simulink model "lic_old"  (R2021b)
settings: Solver=VariableStepAuto  StartTime=0.0  StopTime=10.0  RelTol=1e-3
undefined symbols (not defined in the file): C_TICK_TIME_S, ENUM_LANEQUALITY_HIGH, ENUM_LANEQUALITY_MEDIUM, ENUM_LFCSTATE_DEGRADED, FALSE, KAPP_VehicleWidth_m, KIFO_C1Max4Act_rad, KIFO_C2Max4Act_rat, KIFO_C2Max4Disable_rat, KIFO_C2Max4DisableThr_s, KIFO_Lane4ActThr_s, KIFO_LaneWidthLowThr_m, KIFO_LaneWidthUpThr_m, KIFO_TLCTriggerThrHysis_s, KPER_C0CrossingThr_m, KPER_CalDefaultTLC_s, KPER_CalTLCMax_s, KPER_CalTLCMin_s, KPER_DefaultLaneWidth_m, KPER_LaneWidHoldOnTime_s, KPER_LaneWidRampFinErrThres_m, KPER_LaneWidRampFinTimeThres_s, KPER_LaneWidRampInFalRt_mps, KPER_LaneWidRampInRisRt_mps, KPER_LaneWidRampOutFalRt_mps, KPER_LaneWidRampOutRisRt_mps, KPER_TLCDefaultValue_s, KPER_UseCalTLC_flg, MIFO_TLCThr4LKA_s, TRUE
libraries: hcu_lib x33, simulink x8
(part 2 of 2)

== system lic_old/Lane_Process/LaneCalculation/GenerateLeftLane ==
  VDINR_LaneC0L_m : Inport
  VLIC_EstLaneC0L_m : Inport  Port=2
  VDINR_LaneC1L_rad : Inport  Port=3
  VLIC_EstLaneC1L_rad : Inport  Port=4
  VDINR_LaneC2L_rat : Inport  Port=5
  VLIC_EstLaneC2L_rat : Inport  Port=6
  VDINR_LaneC3L_rat : Inport  Port=7
  VLIC_EstLaneC3L_rat : Inport  Port=8
  VLIC_LeftLaneAvail_flg : Inport  Port=9
  Switch{3,12..14} (4 alike) : Switch  Criteria=u2 ~= 0
  VLIC_LaneC0L_m : Outport
  VLIC_LaneC1L_rad : Outport  Port=2
  VLIC_LaneC2L_rat : Outport  Port=3
  VLIC_LaneC3L_rat : Outport  Port=4
  wires:
  Switch14/1 -> VLIC_LaneC3L_rat/1  "VLIC_LaneC3L_rat"
  VDINR_LaneC0L_m/1 -> Switch3/1
  VDINR_LaneC3L_rat/1 -> Switch14/1
  VLIC_EstLaneC3L_rat/1 -> Switch14/3
  VLIC_LeftLaneAvail_flg/1 -> Switch3/2, Switch12/2, Switch13/2, Switch14/2
  VDINR_LaneC2L_rat/1 -> Switch13/1
  VLIC_EstLaneC2L_rat/1 -> Switch13/3
  Switch13/1 -> VLIC_LaneC2L_rat/1  "VLIC_LaneC2L_rat"
  Switch3/1 -> VLIC_LaneC0L_m/1  "VLIC_LaneC0L_m"
  VDINR_LaneC1L_rad/1 -> Switch12/1
  VLIC_EstLaneC1L_rad/1 -> Switch12/3
  Switch12/1 -> VLIC_LaneC1L_rad/1  "VLIC_LaneC1L_rad"
  VLIC_EstLaneC0L_m/1 -> Switch3/3

== system lic_old/Lane_Process/LaneCalculation/GenerateRightLane ==
  VDINR_LaneC0R_m : Inport
  VLIC_EstLaneC0R_m : Inport  Port=2
  VDINR_LaneC1R_rad : Inport  Port=3
  VLIC_EstLaneC1R_rad : Inport  Port=4
  VDINR_LaneC2R_rat : Inport  Port=5
  VLIC_EstLaneC2R_rat : Inport  Port=6
  VDINR_LaneC3R_rat : Inport  Port=7
  VLIC_EstLaneC3R_rat : Inport  Port=8
  VLIC_RightLaneAvail_flg : Inport  Port=9
  Switch{3,12..14} (4 alike) : Switch  Criteria=u2 ~= 0
  VLIC_LaneC0R_m : Outport
  VLIC_LaneC1R_rad : Outport  Port=2
  VLIC_LaneC2R_rat : Outport  Port=3
  VLIC_LaneC3R_rat : Outport  Port=4
  wires:
  VLIC_EstLaneC0R_m/1 -> Switch3/3
  Switch12/1 -> VLIC_LaneC1R_rad/1  "VLIC_LaneC1R_rad"
  VLIC_EstLaneC1R_rad/1 -> Switch12/3
  VDINR_LaneC1R_rad/1 -> Switch12/1
  Switch3/1 -> VLIC_LaneC0R_m/1  "VLIC_LaneC0R_m"
  Switch13/1 -> VLIC_LaneC2R_rat/1  "VLIC_LaneC2R_rat"
  VLIC_EstLaneC2R_rat/1 -> Switch13/3
  VDINR_LaneC2R_rat/1 -> Switch13/1
  VLIC_RightLaneAvail_flg/1 -> Switch14/2, Switch13/2, Switch12/2, Switch3/2
  Switch14/1 -> VLIC_LaneC3R_rat/1  "VLIC_LaneC3R_rat"
  VLIC_EstLaneC3R_rat/1 -> Switch14/3
  VDINR_LaneC3R_rat/1 -> Switch14/1
  VDINR_LaneC0R_m/1 -> Switch3/1

== system lic_old/Lane_Process/LaneCalculation/LR_Available ==
  VDINR_LaneC0L_m : Inport
  VDINR_LaneC0R_m : Inport  Port=2
  VDINR_LaneC1L_rad : Inport  Port=3
  VDINR_LaneC1R_rad : Inport  Port=4
  VDINR_LaneC2L_rat : Inport  Port=5
  VDINR_LaneC2R_rat : Inport  Port=6
  VDINR_LaneC3L_rat : Inport  Port=7
  VDINR_LaneC3R_rat : Inport  Port=8
  Enable : EnablePort  StatesWhenEnabling=reset
  Add{,1..3} (4 alike) : Sum
  Gain{,1..3} (4 alike) : Gain  Gain=0.5
  VLIC_RLCenterLineC0_m : Outport
  VLIC_RLCenterLineC1_rad : Outport  Port=2
  VLIC_RLCenterLineC2_rat : Outport  Port=3
  VLIC_RLCenterLineC3_rat : Outport  Port=4
  wires:
  Gain3/1 -> VLIC_RLCenterLineC3_rat/1  "VLIC_RLCenterLineC3_rat"
  VDINR_LaneC3R_rat/1 -> Add3/2
  VDINR_LaneC3L_rat/1 -> Add3/1
  Add3/1 -> Gain3/1
  Gain2/1 -> VLIC_RLCenterLineC2_rat/1  "VLIC_RLCenterLineC2_rat"
  VDINR_LaneC2R_rat/1 -> Add2/2
  VDINR_LaneC2L_rat/1 -> Add2/1
  Gain1/1 -> VLIC_RLCenterLineC1_rad/1  "VLIC_RLCenterLineC1_rad"
  Add2/1 -> Gain2/1
  Add1/1 -> Gain1/1
  VDINR_LaneC1R_rad/1 -> Add1/2
  VDINR_LaneC1L_rad/1 -> Add1/1
  Gain/1 -> VLIC_RLCenterLineC0_m/1  "VLIC_RLCenterLineC0_m"
  Add/1 -> Gain/1
  VDINR_LaneC0R_m/1 -> Add/2
  VDINR_LaneC0L_m/1 -> Add/1

== system lic_old/Lane_Process/LaneCalculation/LR_NotAvailable ==
  VLIC_EstLaneC0L_m : Inport
  VLIC_EstLaneC0R_m : Inport  Port=2
  VLIC_EstLaneC1L_rad : Inport  Port=3
  VLIC_EstLaneC1R_rad : Inport  Port=4
  VLIC_EstLaneC2L_rat : Inport  Port=5
  VLIC_EstLaneC2R_rat : Inport  Port=6
  VLIC_EstLaneC3L_rat : Inport  Port=7
  VLIC_EstLaneC3R_rat : Inport  Port=8
  Enable : EnablePort  StatesWhenEnabling=reset
  Add{,1..3} (4 alike) : Sum
  Gain{,1..3} (4 alike) : Gain  Gain=0.5
  VLIC_EstCenterLineC0_m : Outport
  VLIC_EstCenterLineC1_rad : Outport  Port=2
  VLIC_EstCenterLineC2_rat : Outport  Port=3
  VLIC_EstCenterLineC3_rat : Outport  Port=4
  wires:
  Gain3/1 -> VLIC_EstCenterLineC3_rat/1  "VLIC_EstCenterLineC3_rat"
  VLIC_EstLaneC3R_rat/1 -> Add3/2
  VLIC_EstLaneC3L_rat/1 -> Add3/1
  Add3/1 -> Gain3/1
  Gain2/1 -> VLIC_EstCenterLineC2_rat/1  "VLIC_EstCenterLineC2_rat"
  VLIC_EstLaneC2R_rat/1 -> Add2/2
  VLIC_EstLaneC2L_rat/1 -> Add2/1
  Gain1/1 -> VLIC_EstCenterLineC1_rad/1  "VLIC_EstCenterLineC1_rad"
  Add2/1 -> Gain2/1
  Add1/1 -> Gain1/1
  VLIC_EstLaneC1R_rad/1 -> Add1/2
  VLIC_EstLaneC1L_rad/1 -> Add1/1
  Gain/1 -> VLIC_EstCenterLineC0_m/1  "VLIC_EstCenterLineC0_m"
  Add/1 -> Gain/1
  VLIC_EstLaneC0R_m/1 -> Add/2
  VLIC_EstLaneC0L_m/1 -> Add/1

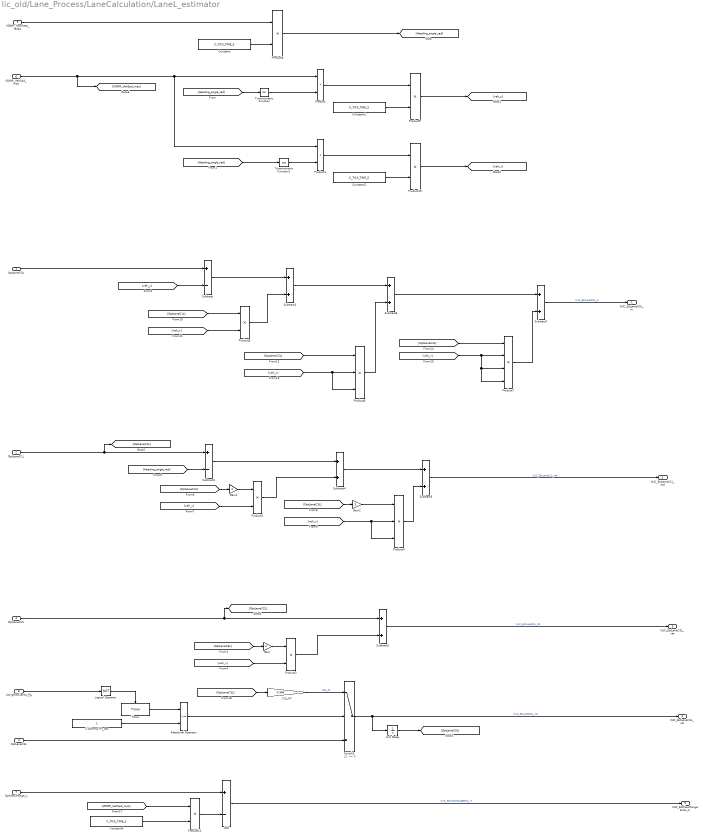
== system lic_old/Lane_Process/LaneCalculation/LaneL_estimator ==
  OptLaneC0L : Inport
  OptLaneC1L : Inport  Port=2
  OptLaneC2L : Inport  Port=3
  OptLaneC3L : Inport  Port=4
  VDINR_YawRate_radps : Inport  Port=5
  VDINR_VehSpd_mps : Inport  Port=6
  OptViewRange_L : Inport  Port=7
  UsingRawLaneL_flg : Inport  Port=8
  Add : Sum  Inputs=+-
  C3LRampThr_sec : Constant  OutDataTypeStr=single
  C3L_FF : Gain  Gain=0.994
  Constant{,1..2,4} (4 alike) : Constant  Value=C_TICK_TIME_S
  Gain : Gain  Gain=3
  Gain1 : Gain  Gain=2
  Gain2 : Gain  Gain=3
  Logical Operator : Logic  Operator=NOT  AllPortsSameDT=off  OutDataTypeStr=boolean
  Product{,1..3,5,8..10,12} (9 alike) : Product
  Product4 : Product  Inputs=3
  Product6 : Product  Inputs=3
  Product7 : Product  Inputs=4
  Relational Operator : RelationalOperator  OutDataTypeStr=boolean  RndMeth=Nearest
  Subtract : Sum  Inputs=+-
  Subtract{1..2,4..7} (6 alike) : Sum
  Subtract3 : Sum  Inputs=+-
  Switch2 : Switch  Criteria=u2 ~= 0
  Timer : hcu_lib/Timer  SystemSampleTime=-1  VariantActivationTime=update diagram  Latency=0  AutoFrameSizeCalculation=off
  Trigonometric Function : Trigonometry
  Trigonometric Function1 : Trigonometry  Operator=cos
  Unit Delay : UnitDelay  SampleTime=-1  HasFrameUpgradeWarning=on
  VLIC_EstLaneC0L_m : Outport
  VLIC_EstLaneC1L_rad : Outport  Port=2
  VLIC_EstLaneC2L_rat : Outport  Port=3
  VLIC_EstLaneC3L_rat : Outport  Port=4
  VLIC_EstViewRangeEndL_m : Outport  Port=5
  wires:
  Product8/1 -> [Heading_angle_rad]
  Unit Delay/1 -> [OptLaneC3L]
  Logical Operator/1 -> Timer/Enable
  C3L_FF/1 -> Switch2/1  "C3L_FF"
  [OptLaneC3L] -> C3L_FF/1
  Switch2/1 -> VLIC_EstLaneC3L_rat/1, Unit Delay/1  "VLIC_EstLaneC3L_rat"
  OptLaneC3L/1 -> Switch2/3
  Relational Operator/1 -> Switch2/2
  C3LRampThr_sec/1 -> Relational Operator/2
  Timer/1 -> Relational Operator/1
  UsingRawLaneL_flg/1 -> Logical Operator/1
  Constant4/1 -> Product12/2
  Add/1 -> VLIC_EstViewRangeEndL_m/1  "VLIC_EstViewRangeEndL_m"
  Product12/1 -> Add/2
  [VDINR_VehSpd_mps] -> Product12/1
  OptViewRange_L/1 -> Add/1
  VDINR_YawRate_radps/1 -> Product8/1
  Product1/1 -> Product10/1
  Constant2/1 -> Product10/2
  Product/1 -> Product9/1
  Constant1/1 -> Product9/2
  Constant/1 -> Product8/2
  Subtract7/1 -> VLIC_EstLaneC0L_m/1  "VLIC_EstLaneC0L_m"
  Product7/1 -> Subtract7/2
  [veh_x] -> Product7/3, Product7/4, Product7/2
  [OptLaneC3L] -> Product7/1
  Subtract6/1 -> Subtract7/1
  Product6/1 -> Subtract6/2
  [veh_x] -> Product6/3, Product6/2
  [OptLaneC2L] -> Product6/1
  Subtract1/1 -> Subtract6/1
  Product5/1 -> Subtract1/2
  [veh_x] -> Product5/2
  [OptLaneC1L] -> Product5/1
  Subtract5/1 -> VLIC_EstLaneC1L_rad/1  "VLIC_EstLaneC1L_rad"
  Product4/1 -> Subtract5/2
  [veh_x] -> Product4/2, Product4/3
  Gain2/1 -> Product4/1
  [OptLaneC3L] -> Gain2/1
  Subtract4/1 -> Subtract5/1
  Product3/1 -> Subtract4/2
  [veh_x] -> Product3/2
  Gain1/1 -> Product3/1
  [OptLaneC2L] -> Gain1/1
  Subtract3/1 -> Subtract4/1
  [Heading_angle_rad] -> Subtract3/2
  OptLaneC1L/1 -> Subtract3/1, [OptLaneC1L]
  Subtract2/1 -> VLIC_EstLaneC2L_rat/1  "VLIC_EstLaneC2L_rat"
  [veh_x] -> Product2/2
  Gain/1 -> Product2/1
  [OptLaneC3L] -> Gain/1
  Product2/1 -> Subtract2/2
  OptLaneC2L/1 -> Subtract2/1, [OptLaneC2L]
  Subtract/1 -> Subtract1/1
  [veh_y] -> Subtract/2
  OptLaneC0L/1 -> Subtract/1
  Product10/1 -> [veh_x]
  Trigonometric Function1/1 -> Product1/2
  [Heading_angle_rad] -> Trigonometric Function1/1
  Product9/1 -> [veh_y]
  Trigonometric Function/1 -> Product/2
  [Heading_angle_rad] -> Trigonometric Function/1
  VDINR_VehSpd_mps/1 -> Product/1, Product1/1, [VDINR_VehSpd_mps]

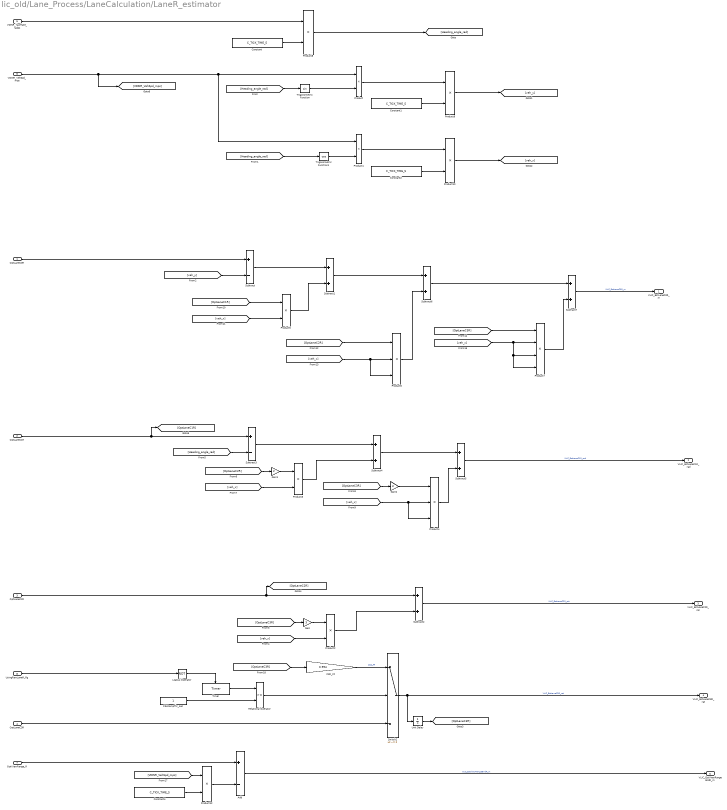
== system lic_old/Lane_Process/LaneCalculation/LaneR_estimator ==
  OptLaneC0R : Inport
  OptLaneC1R : Inport  Port=2
  OptLaneC2R : Inport  Port=3
  OptLaneC3R : Inport  Port=4
  VDINR_YawRate_radps : Inport  Port=5
  VDINR_VehSpd_mps : Inport  Port=6
  OptViewRange_R : Inport  Port=7
  UsingRawLaneR_flg : Inport  Port=8
  Add : Sum  Inputs=+-
  C3LRampThr_sec : Constant  OutDataTypeStr=single
  C3R_FF : Gain  Gain=0.994
  Constant{,1..2,4} (4 alike) : Constant  Value=C_TICK_TIME_S
  Gain : Gain  Gain=3
  Gain1 : Gain  Gain=2
  Gain2 : Gain  Gain=3
  Logical Operator : Logic  Operator=NOT  AllPortsSameDT=off  OutDataTypeStr=boolean
  Product{,1..3,5,8..10,12} (9 alike) : Product
  Product4 : Product  Inputs=3
  Product6 : Product  Inputs=3
  Product7 : Product  Inputs=4
  Relational Operator : RelationalOperator  OutDataTypeStr=boolean  RndMeth=Nearest
  Subtract : Sum  Inputs=+-
  Subtract{1..2,4..7} (6 alike) : Sum
  Subtract3 : Sum  Inputs=+-
  Switch2 : Switch  Criteria=u2 ~= 0
  Timer : hcu_lib/Timer  SystemSampleTime=-1  VariantActivationTime=update diagram  Latency=0  AutoFrameSizeCalculation=off
  Trigonometric Function : Trigonometry
  Trigonometric Function1 : Trigonometry  Operator=cos
  Unit Delay : UnitDelay  SampleTime=-1  HasFrameUpgradeWarning=on
  VLIC_EstLaneC0R_m : Outport
  VLIC_EstLaneC1R_rad : Outport  Port=2
  VLIC_EstLaneC2R_rat : Outport  Port=3
  VLIC_EstLaneC3R_rat : Outport  Port=4
  VLIC_EstViewRangeEndR_m : Outport  Port=5
  wires:
  Unit Delay/1 -> [OptLaneC3R]
  Logical Operator/1 -> Timer/Enable
  OptLaneC3R/1 -> Switch2/3
  C3R_FF/1 -> Switch2/1  "C3R_FF"
  [OptLaneC3R] -> C3R_FF/1
  Switch2/1 -> VLIC_EstLaneC3R_rat/1, Unit Delay/1  "VLIC_EstLaneC3R_rat"
  Relational Operator/1 -> Switch2/2
  C3LRampThr_sec/1 -> Relational Operator/2
  Timer/1 -> Relational Operator/1
  UsingRawLaneR_flg/1 -> Logical Operator/1
  VDINR_VehSpd_mps/1 -> [VDINR_VehSpd_mps], Product1/1, Product/1
  [Heading_angle_rad] -> Trigonometric Function/1
  Trigonometric Function/1 -> Product/2
  Product9/1 -> [veh_y]
  [Heading_angle_rad] -> Trigonometric Function1/1
  Trigonometric Function1/1 -> Product1/2
  Product10/1 -> [veh_x]
  OptLaneC0R/1 -> Subtract/1
  [veh_y] -> Subtract/2
  Subtract/1 -> Subtract1/1
  OptLaneC2R/1 -> [OptLaneC2R], Subtract2/1
  Product2/1 -> Subtract2/2
  [OptLaneC3R] -> Gain/1
  Gain/1 -> Product2/1
  [veh_x] -> Product2/2
  Subtract2/1 -> VLIC_EstLaneC2R_rat/1  "VLIC_EstLaneC2R_rat"
  OptLaneC1R/1 -> [OptLaneC1R], Subtract3/1
  [Heading_angle_rad] -> Subtract3/2
  Subtract3/1 -> Subtract4/1
  [OptLaneC2R] -> Gain1/1
  Gain1/1 -> Product3/1
  [veh_x] -> Product3/2
  Product3/1 -> Subtract4/2
  Subtract4/1 -> Subtract5/1
  [OptLaneC3R] -> Gain2/1
  Gain2/1 -> Product4/1
  [veh_x] -> Product4/3, Product4/2
  Product4/1 -> Subtract5/2
  Subtract5/1 -> VLIC_EstLaneC1R_rad/1  "VLIC_EstLaneC1R_rad"
  [OptLaneC1R] -> Product5/1
  [veh_x] -> Product5/2
  Product5/1 -> Subtract1/2
  Subtract1/1 -> Subtract6/1
  [OptLaneC2R] -> Product6/1
  [veh_x] -> Product6/2, Product6/3
  Product6/1 -> Subtract6/2
  Subtract6/1 -> Subtract7/1
  [OptLaneC3R] -> Product7/1
  [veh_x] -> Product7/2, Product7/4, Product7/3
  Product7/1 -> Subtract7/2
  Subtract7/1 -> VLIC_EstLaneC0R_m/1  "VLIC_EstLaneC0R_m"
  Constant/1 -> Product8/2
  Constant1/1 -> Product9/2
  Product/1 -> Product9/1
  Constant2/1 -> Product10/2
  Product1/1 -> Product10/1
  VDINR_YawRate_radps/1 -> Product8/1
  Product8/1 -> [Heading_angle_rad]
  OptViewRange_R/1 -> Add/1
  [VDINR_VehSpd_mps] -> Product12/1
  Constant4/1 -> Product12/2
  Product12/1 -> Add/2
  Add/1 -> VLIC_EstViewRangeEndR_m/1  "VLIC_EstViewRangeEndR_m"

== system lic_old/Lane_Process/LaneCalculation/LaneResidual_Calculation ==
  VLIC_EstViewRangeEndL_m : Inport
  VDINR_VehSpd_mps : Inport  Port=2
  VLIC_EstViewRangeEndR_m : Inport  Port=3
  Constant6 : Constant  Value=3  OutDataTypeStr=single
  Constant7 : Constant  Value=3  OutDataTypeStr=single
  Saturation1 : Saturate  UpperLimit=3  LowerLimit=0
      settings: AttributesFormatString=upper = %<UpperLimit>\nlower = %<LowerLimit>
  Saturation2 : Saturate  UpperLimit=3  LowerLimit=0
      settings: AttributesFormatString=upper = %<UpperLimit>\nlower = %<LowerLimit>
  divide : hcu_lib/divide
  divide1 : hcu_lib/divide
  VLIC_ResidualLaneL_s : Outport
  VLIC_ResidualLaneR_s : Outport  Port=2
  wires:
  Saturation2/1 -> VLIC_ResidualLaneR_s/1  "VLIC_ResidualLaneR_s"
  Saturation1/1 -> VLIC_ResidualLaneL_s/1  "VLIC_ResidualLaneL_s"
  divide1/1 -> Saturation2/1
  Constant7/1 -> divide1/3
  VDINR_VehSpd_mps/1 -> divide/2, divide1/2
  VLIC_EstViewRangeEndR_m/1 -> divide1/1
  Constant6/1 -> divide/3
  VLIC_EstViewRangeEndL_m/1 -> divide/1
  divide/1 -> Saturation1/1

== system lic_old/Lane_Process/LaneCalculation/LaneWidth ==
  VLIC_LeftLaneAvail_flg : Inport
  VLIC_RightLaneAvail_flg : Inport  Port=2
  VLIC_LaneC0L_m : Inport  Port=3
  VLIC_LaneC0R_m : Inport  Port=4
  Add : Sum  Inputs=+-
  Delay : Delay  DelayLength=1  InitialCondition=KPER_DefaultLaneWidth_m
  KPER_DefaultLaneWidth_m : Constant  Value=KPER_DefaultLaneWidth_m
  KPER_LaneWidHoldOnTime_s : Constant  Value=KPER_LaneWidHoldOnTime_s
  KPER_LaneWidRampFinErrThres_m : Constant  Value=KPER_LaneWidRampFinErrThres_m
  KPER_LaneWidRampFinTimeThres_s : Constant  Value=KPER_LaneWidRampFinTimeThres_s
  KPER_LaneWidRampInFalRt_mps : Constant  Value=KPER_LaneWidRampInFalRt_mps
  KPER_LaneWidRampInRisRt_mps : Constant  Value=KPER_LaneWidRampInRisRt_mps
  KPER_LaneWidRampOutFalRt_mps : Constant  Value=KPER_LaneWidRampOutFalRt_mps
  KPER_LaneWidRampOutRisRt_mps : Constant  Value=KPER_LaneWidRampOutRisRt_mps
  Logical Operator : Logic  Operator=OR  AllPortsSameDT=off  OutDataTypeStr=boolean
  Logical Operator1 : Logic  Operator=NOT  AllPortsSameDT=off  OutDataTypeStr=boolean
  Logical Operator2 : Logic  Operator=NOT  AllPortsSameDT=off  OutDataTypeStr=boolean
  RampInRampOut : hcu_lib/RampInRampOut  SystemSampleTime=-1  VariantActivationTime=update diagram  Latency=0  AutoFrameSizeCalculation=off
  Relational Operator2 : RelationalOperator  OutDataTypeStr=boolean  RndMeth=Nearest
  Switch2 : Switch  Criteria=u2 ~= 0
  Timer : hcu_lib/Timer  SystemSampleTime=-1  VariantActivationTime=update diagram  Latency=0  AutoFrameSizeCalculation=off
  VLIC_LaneWidth_m : Outport
  wires:
  VLIC_RightLaneAvail_flg/1 -> Logical Operator2/1
  VLIC_LeftLaneAvail_flg/1 -> Logical Operator1/1
  KPER_LaneWidHoldOnTime_s/1 -> Relational Operator2/2
  Timer/1 -> Relational Operator2/1
  Relational Operator2/1 -> RampInRampOut/3
  RampInRampOut/1 -> VLIC_LaneWidth_m/1, Delay/1  "VLIC_LaneWidth_m"
  KPER_LaneWidRampFinTimeThres_s/1 -> RampInRampOut/9
  KPER_LaneWidRampFinErrThres_m/1 -> RampInRampOut/8
  KPER_LaneWidRampOutRisRt_mps/1 -> RampInRampOut/6
  KPER_LaneWidRampOutFalRt_mps/1 -> RampInRampOut/7
  KPER_LaneWidRampInFalRt_mps/1 -> RampInRampOut/5
  KPER_LaneWidRampInRisRt_mps/1 -> RampInRampOut/4
  Logical Operator/1 -> Timer/Enable, Switch2/2
  KPER_DefaultLaneWidth_m/1 -> RampInRampOut/2
  Delay/1 -> Switch2/1
  Switch2/1 -> RampInRampOut/1
  Logical Operator1/1 -> Logical Operator/1
  Logical Operator2/1 -> Logical Operator/2
  VLIC_LaneC0L_m/1 -> Add/1
  Add/1 -> Switch2/3
  VLIC_LaneC0R_m/1 -> Add/2

== system lic_old/Lane_Process/LaneCalculation/OnlyL_Available ==
  VLIC_LaneWidth_m : Inport
  VDINR_LaneC0L_m : Inport  Port=2
  VDINR_LaneC1L_rad : Inport  Port=3
  VDINR_LaneC2L_rat : Inport  Port=4
  VDINR_LaneC3L_rat : Inport  Port=5
  Enable : EnablePort  StatesWhenEnabling=reset
  Add : Sum  Inputs=-+
  Add1 : Sum
  Data Type Conversion : DataTypeConversion  OutDataTypeStr=single
  Data Type Conversion1 : DataTypeConversion  OutDataTypeStr=single
  Data Type Conversion2 : DataTypeConversion  OutDataTypeStr=single
  Gain : Gain  Gain=0.5
  VLIC_LCenterLineC0_m : Outport
  VLIC_LCenterLineC1_rad : Outport  Port=2
  VLIC_LCenterLineC2_rat : Outport  Port=3
  VLIC_LCenterLineC3_rat : Outport  Port=4
  wires:
  Data Type Conversion/1 -> VLIC_LCenterLineC1_rad/1  "VLIC_LCenterLineC1_rad"
  Data Type Conversion2/1 -> VLIC_LCenterLineC3_rat/1  "VLIC_LCenterLineC3_rat"
  Data Type Conversion1/1 -> VLIC_LCenterLineC2_rat/1  "VLIC_LCenterLineC2_rat"
  Gain/1 -> VLIC_LCenterLineC0_m/1  "VLIC_LCenterLineC0_m"
  Add1/1 -> Gain/1
  Add/1 -> Add1/1
  VDINR_LaneC3L_rat/1 -> Data Type Conversion2/1
  VDINR_LaneC2L_rat/1 -> Data Type Conversion1/1
  VDINR_LaneC0L_m/1 -> Add/2, Add1/2
  VLIC_LaneWidth_m/1 -> Add/1
  VDINR_LaneC1L_rad/1 -> Data Type Conversion/1

== system lic_old/Lane_Process/LaneCalculation/OnlyR_Available ==
  VLIC_LaneWidth_m : Inport
  VDINR_LaneC0R_m : Inport  Port=2
  VDINR_LaneC1R_rad : Inport  Port=3
  VDINR_LaneC2R_rat : Inport  Port=4
  VDINR_LaneC3R_rat : Inport  Port=5
  Enable : EnablePort  StatesWhenEnabling=reset
  Add : Sum
  Add1 : Sum
  Data Type Conversion : DataTypeConversion  OutDataTypeStr=single
  Data Type Conversion1 : DataTypeConversion  OutDataTypeStr=single
  Data Type Conversion2 : DataTypeConversion  OutDataTypeStr=single
  Gain : Gain  Gain=0.5
  VLIC_RCenterLineC0_m : Outport
  VLIC_RCenterLineC1_rad : Outport  Port=2
  VLIC_RCenterLineC2_rat : Outport  Port=3
  VLIC_RCenterLineC3_rat : Outport  Port=4
  wires:
  Data Type Conversion2/1 -> VLIC_RCenterLineC3_rat/1  "VLIC_RCenterLineC3_rat"
  Data Type Conversion1/1 -> VLIC_RCenterLineC2_rat/1  "VLIC_RCenterLineC2_rat"
  Data Type Conversion/1 -> VLIC_RCenterLineC1_rad/1  "VLIC_RCenterLineC1_rad"
  Gain/1 -> VLIC_RCenterLineC0_m/1  "VLIC_RCenterLineC0_m"
  Add1/1 -> Gain/1
  Add/1 -> Add1/1
  VDINR_LaneC1R_rad/1 -> Data Type Conversion/1
  VLIC_LaneWidth_m/1 -> Add/1
  VDINR_LaneC0R_m/1 -> Add/2, Add1/2
  VDINR_LaneC2R_rat/1 -> Data Type Conversion1/1
  VDINR_LaneC3R_rat/1 -> Data Type Conversion2/1

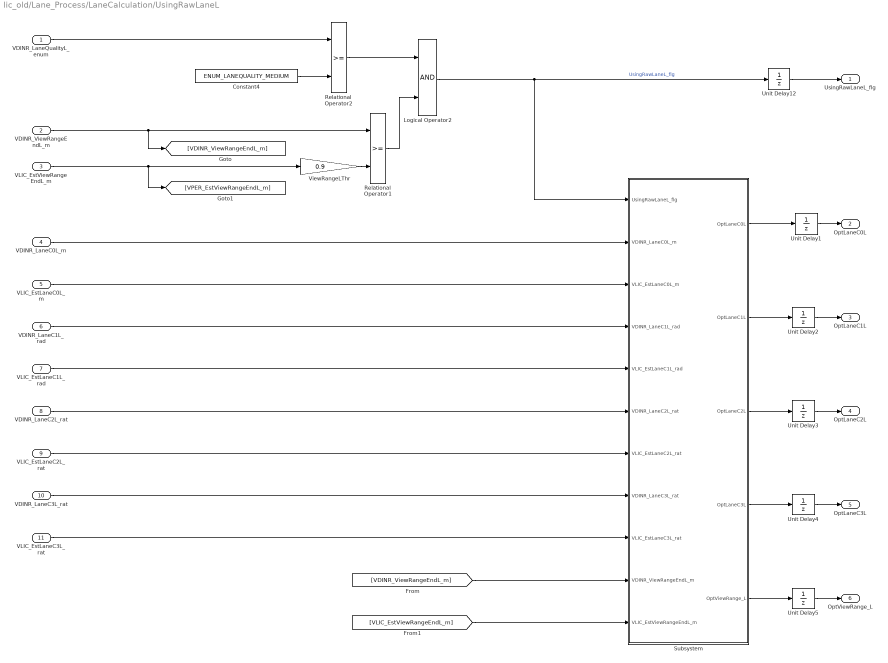
== system lic_old/Lane_Process/LaneCalculation/UsingRawLaneL ==
  VDINR_LaneQualityL_enum : Inport
  VDINR_ViewRangeEndL_m : Inport  Port=2
  VLIC_EstViewRangeEndL_m : Inport  Port=3
  VDINR_LaneC0L_m : Inport  Port=4
  VLIC_EstLaneC0L_m : Inport  Port=5
  VDINR_LaneC1L_rad : Inport  Port=6
  VLIC_EstLaneC1L_rad : Inport  Port=7
  VDINR_LaneC2L_rat : Inport  Port=8
  VLIC_EstLaneC2L_rat : Inport  Port=9
  VDINR_LaneC3L_rat : Inport  Port=10
  VLIC_EstLaneC3L_rat : Inport  Port=11
  Constant4 : Constant  Value=ENUM_LANEQUALITY_MEDIUM
  Logical Operator2 : Logic  AllPortsSameDT=off  OutDataTypeStr=boolean
  Relational Operator1 : RelationalOperator  OutDataTypeStr=boolean  RndMeth=Nearest
  Relational Operator2 : RelationalOperator  OutDataTypeStr=boolean  RndMeth=Nearest
  Subsystem : Subsystem
  Unit Delay{1..5,12} (6 alike) : UnitDelay  SampleTime=-1  HasFrameUpgradeWarning=on
  ViewRangeLThr : Gain  Gain=0.9
  UsingRawLaneL_flg : Outport
  OptLaneC0L : Outport  Port=2
  OptLaneC1L : Outport  Port=3
  OptLaneC2L : Outport  Port=4
  OptLaneC3L : Outport  Port=5
  OptViewRange_L : Outport  Port=6
  wires:
  Subsystem/5(OptViewRange_L) -> Unit Delay5/1
  Subsystem/4(OptLaneC3L) -> Unit Delay4/1
  Subsystem/3(OptLaneC2L) -> Unit Delay3/1
  Subsystem/2(OptLaneC1L) -> Unit Delay2/1
  Subsystem/1(OptLaneC0L) -> Unit Delay1/1
  [VDINR_ViewRangeEndL_m] -> Subsystem/10(VDINR_ViewRangeEndL_m)
  [VLIC_EstViewRangeEndL_m] -> Subsystem/11(VLIC_EstViewRangeEndL_m)
  VLIC_EstLaneC3L_rat/1 -> Subsystem/9(VLIC_EstLaneC3L_rat)
  VDINR_LaneC3L_rat/1 -> Subsystem/8(VDINR_LaneC3L_rat)
  VLIC_EstLaneC2L_rat/1 -> Subsystem/7(VLIC_EstLaneC2L_rat)
  VDINR_LaneC2L_rat/1 -> Subsystem/6(VDINR_LaneC2L_rat)
  VLIC_EstLaneC1L_rad/1 -> Subsystem/5(VLIC_EstLaneC1L_rad)
  VDINR_LaneC1L_rad/1 -> Subsystem/4(VDINR_LaneC1L_rad)
  VLIC_EstLaneC0L_m/1 -> Subsystem/3(VLIC_EstLaneC0L_m)
  VDINR_LaneC0L_m/1 -> Subsystem/2(VDINR_LaneC0L_m)
  Logical Operator2/1 -> Unit Delay12/1, Subsystem/1(UsingRawLaneL_flg)  "UsingRawLaneL_flg"
  VDINR_LaneQualityL_enum/1 -> Relational Operator2/1
  Constant4/1 -> Relational Operator2/2
  Relational Operator2/1 -> Logical Operator2/1
  VDINR_ViewRangeEndL_m/1 -> Relational Operator1/1, [VDINR_ViewRangeEndL_m]
  VLIC_EstViewRangeEndL_m/1 -> ViewRangeLThr/1, [VPER_EstViewRangeEndL_m]
  ViewRangeLThr/1 -> Relational Operator1/2
  Relational Operator1/1 -> Logical Operator2/2
  Unit Delay12/1 -> UsingRawLaneL_flg/1
  Unit Delay1/1 -> OptLaneC0L/1
  Unit Delay2/1 -> OptLaneC1L/1
  Unit Delay3/1 -> OptLaneC2L/1
  Unit Delay4/1 -> OptLaneC3L/1
  Unit Delay5/1 -> OptViewRange_L/1

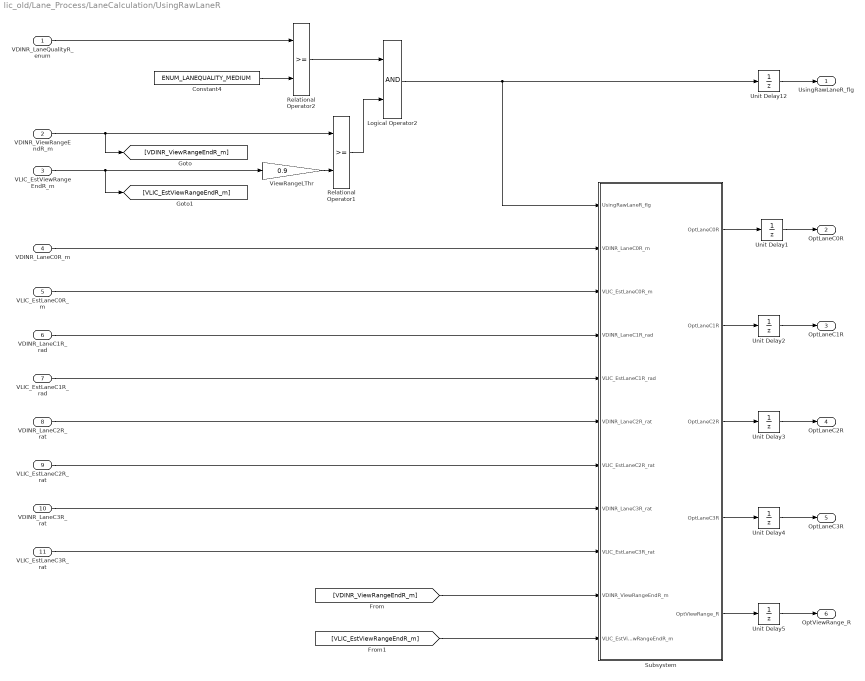
== system lic_old/Lane_Process/LaneCalculation/UsingRawLaneR ==
  VDINR_LaneQualityR_enum : Inport
  VDINR_ViewRangeEndR_m : Inport  Port=2
  VLIC_EstViewRangeEndR_m : Inport  Port=3
  VDINR_LaneC0R_m : Inport  Port=4
  VLIC_EstLaneC0R_m : Inport  Port=5
  VDINR_LaneC1R_rad : Inport  Port=6
  VLIC_EstLaneC1R_rad : Inport  Port=7
  VDINR_LaneC2R_rat : Inport  Port=8
  VLIC_EstLaneC2R_rat : Inport  Port=9
  VDINR_LaneC3R_rat : Inport  Port=10
  VLIC_EstLaneC3R_rat : Inport  Port=11
  Constant4 : Constant  Value=ENUM_LANEQUALITY_MEDIUM
  Logical Operator2 : Logic  AllPortsSameDT=off  OutDataTypeStr=boolean
  Relational Operator1 : RelationalOperator  OutDataTypeStr=boolean  RndMeth=Nearest
  Relational Operator2 : RelationalOperator  OutDataTypeStr=boolean  RndMeth=Nearest
  Subsystem : Subsystem
  Unit Delay{1..5,12} (6 alike) : UnitDelay  SampleTime=-1  HasFrameUpgradeWarning=on
  ViewRangeLThr : Gain  Gain=0.9
  UsingRawLaneR_flg : Outport
  OptLaneC0R : Outport  Port=2
  OptLaneC1R : Outport  Port=3
  OptLaneC2R : Outport  Port=4
  OptLaneC3R : Outport  Port=5
  OptViewRange_R : Outport  Port=6
  wires:
  Subsystem/5(OptViewRange_R) -> Unit Delay5/1
  Subsystem/4(OptLaneC3R) -> Unit Delay4/1
  Subsystem/3(OptLaneC2R) -> Unit Delay3/1
  Subsystem/2(OptLaneC1R) -> Unit Delay2/1
  Subsystem/1(OptLaneC0R) -> Unit Delay1/1
  [VDINR_ViewRangeEndR_m] -> Subsystem/10(VDINR_ViewRangeEndR_m)
  [VLIC_EstViewRangeEndR_m] -> Subsystem/11(VLIC_EstViewRangeEndR_m)
  VLIC_EstLaneC3R_rat/1 -> Subsystem/9(VLIC_EstLaneC3R_rat)
  VDINR_LaneC3R_rat/1 -> Subsystem/8(VDINR_LaneC3R_rat)
  VLIC_EstLaneC2R_rat/1 -> Subsystem/7(VLIC_EstLaneC2R_rat)
  VDINR_LaneC2R_rat/1 -> Subsystem/6(VDINR_LaneC2R_rat)
  VLIC_EstLaneC1R_rad/1 -> Subsystem/5(VLIC_EstLaneC1R_rad)
  VDINR_LaneC1R_rad/1 -> Subsystem/4(VDINR_LaneC1R_rad)
  VLIC_EstLaneC0R_m/1 -> Subsystem/3(VLIC_EstLaneC0R_m)
  VDINR_LaneC0R_m/1 -> Subsystem/2(VDINR_LaneC0R_m)
  Logical Operator2/1 -> Unit Delay12/1, Subsystem/1(UsingRawLaneR_flg)
  VDINR_LaneQualityR_enum/1 -> Relational Operator2/1
  Constant4/1 -> Relational Operator2/2
  Relational Operator2/1 -> Logical Operator2/1
  VDINR_ViewRangeEndR_m/1 -> Relational Operator1/1, [VDINR_ViewRangeEndR_m]
  VLIC_EstViewRangeEndR_m/1 -> ViewRangeLThr/1, [VLIC_EstViewRangeEndR_m]
  ViewRangeLThr/1 -> Relational Operator1/2
  Relational Operator1/1 -> Logical Operator2/2
  Unit Delay12/1 -> UsingRawLaneR_flg/1
  Unit Delay1/1 -> OptLaneC0R/1
  Unit Delay2/1 -> OptLaneC1R/1
  Unit Delay3/1 -> OptLaneC2R/1
  Unit Delay4/1 -> OptLaneC3R/1
  Unit Delay5/1 -> OptViewRange_R/1

== system lic_old/Lane_Process/LaneCalculation/Using_estimator_LeftLane ==
  VDINR_LaneQualityL_enum : Inport
  VDINR_ViewRangeEndL_m : Inport  Port=2
  VLIC_EstViewRangeEndL_m : Inport  Port=3
  Constant6 : Constant  Value=ENUM_LANEQUALITY_MEDIUM
  Logical Operator4 : Logic  AllPortsSameDT=off  OutDataTypeStr=boolean
  Relational Operator5 : RelationalOperator  OutDataTypeStr=boolean  RndMeth=Nearest
  Relational Operator6 : RelationalOperator  OutDataTypeStr=boolean  RndMeth=Nearest
  ViewRangeL : Gain  Gain=0.5
  VLIC_LeftLaneAvail_flg : Outport
  wires:
  VDINR_ViewRangeEndL_m/1 -> Relational Operator5/1
  Constant6/1 -> Relational Operator6/2
  VDINR_LaneQualityL_enum/1 -> Relational Operator6/1
  VLIC_EstViewRangeEndL_m/1 -> ViewRangeL/1
  Relational Operator5/1 -> Logical Operator4/2  "VRTiming_L"
  ViewRangeL/1 -> Relational Operator5/2
  Logical Operator4/1 -> VLIC_LeftLaneAvail_flg/1  "VLIC_LeftLaneAvail_flg"
  Relational Operator6/1 -> Logical Operator4/1

== system lic_old/Lane_Process/LaneCalculation/Using_estimator_RightLane ==
  VDINR_LaneQualityR_enum : Inport
  VDINR_ViewRangeEndR_m : Inport  Port=2
  VLIC_EstViewRangeEndR_m : Inport  Port=3
  Constant7 : Constant  Value=ENUM_LANEQUALITY_MEDIUM
  Logical Operator5 : Logic  AllPortsSameDT=off  OutDataTypeStr=boolean
  Relational Operator7 : RelationalOperator  OutDataTypeStr=boolean  RndMeth=Nearest
  Relational Operator8 : RelationalOperator  OutDataTypeStr=boolean  RndMeth=Nearest
  ViewRangeR : Gain  Gain=0.5
  VLIC_RightLaneAvail_flg : Outport
  wires:
  Logical Operator5/1 -> VLIC_RightLaneAvail_flg/1  "VLIC_RightLaneAvail_flg"
  Relational Operator8/1 -> Logical Operator5/1
  Relational Operator7/1 -> Logical Operator5/2  "VRTiming_R"
  VLIC_EstViewRangeEndR_m/1 -> ViewRangeR/1
  Constant7/1 -> Relational Operator8/2
  VDINR_LaneQualityR_enum/1 -> Relational Operator8/1
  ViewRangeR/1 -> Relational Operator7/2
  VDINR_ViewRangeEndR_m/1 -> Relational Operator7/1

== system lic_old/Lane_Process/LaneCalculation/C1L_Bias/Forgetting_factor ==
  C1LBias_new : Inport
  Enable : EnablePort
  FF : Stateflow chart  TreatAsAtomicUnit=on
  Forget_factor : Constant  Value=0.99933  OutDataTypeStr=single
  Terminator : Terminator
  C1L_Bias : Outport
  wires:
  Forget_factor/1 -> FF/2(Forget_Factor)
  FF/2(P_L) -> Terminator/1
  FF/1(C1L_Bias) -> C1L_Bias/1
  C1LBias_new/1 -> FF/1(C1LBias_new)

== system lic_old/Lane_Process/LaneCalculation/C1R_Bias/Forgetting_factor ==
  C1RBias_new : Inport
  Enable : EnablePort
  FF : Stateflow chart  TreatAsAtomicUnit=on
  Forget_factor : Constant  Value=0.99933  OutDataTypeStr=single
  Terminator : Terminator
  C1R_Bias : Outport
  wires:
  Forget_factor/1 -> FF/2(Forget_Factor)
  FF/2(P_R) -> Terminator/1
  FF/1(C1R_Bias) -> C1R_Bias/1
  C1RBias_new/1 -> FF/1(C1RBias_new)

== system lic_old/Lane_Process/LaneCalculation/UsingRawLaneL/Subsystem ==
  UsingRawLaneL_flg : Inport
  VDINR_LaneC0L_m : Inport  Port=2
  VLIC_EstLaneC0L_m : Inport  Port=3
  VDINR_LaneC1L_rad : Inport  Port=4
  VLIC_EstLaneC1L_rad : Inport  Port=5
  VDINR_LaneC2L_rat : Inport  Port=6
  VLIC_EstLaneC2L_rat : Inport  Port=7
  VDINR_LaneC3L_rat : Inport  Port=8
  VLIC_EstLaneC3L_rat : Inport  Port=9
  VDINR_ViewRangeEndL_m : Inport  Port=10
  VLIC_EstViewRangeEndL_m : Inport  Port=11
  Switch{1,4..7} (5 alike) : Switch  Criteria=u2 ~= 0
  OptLaneC0L : Outport
  OptLaneC1L : Outport  Port=2
  OptLaneC2L : Outport  Port=3
  OptLaneC3L : Outport  Port=4
  OptViewRange_L : Outport  Port=5
  wires:
  VDINR_LaneC0L_m/1 -> Switch4/1
  VLIC_EstLaneC0L_m/1 -> Switch4/3
  VDINR_LaneC1L_rad/1 -> Switch5/1
  VLIC_EstLaneC1L_rad/1 -> Switch5/3
  VDINR_LaneC2L_rat/1 -> Switch6/1
  VLIC_EstLaneC2L_rat/1 -> Switch6/3
  Switch6/1 -> OptLaneC2L/1  "OptLaneC2L"
  VDINR_LaneC3L_rat/1 -> Switch7/1
  VLIC_EstLaneC3L_rat/1 -> Switch7/3
  Switch7/1 -> OptLaneC3L/1  "OptLaneC3L"
  Switch4/1 -> OptLaneC0L/1  "OptLaneC0L"
  Switch5/1 -> OptLaneC1L/1  "OptLaneC1L"
  VDINR_ViewRangeEndL_m/1 -> Switch1/1
  UsingRawLaneL_flg/1 -> Switch4/2, Switch6/2, Switch7/2, Switch1/2, Switch5/2
  VLIC_EstViewRangeEndL_m/1 -> Switch1/3
  Switch1/1 -> OptViewRange_L/1  "OptViewRange_L"

== system lic_old/Lane_Process/LaneCalculation/UsingRawLaneR/Subsystem ==
  UsingRawLaneR_flg : Inport
  VDINR_LaneC0R_m : Inport  Port=2
  VLIC_EstLaneC0R_m : Inport  Port=3
  VDINR_LaneC1R_rad : Inport  Port=4
  VLIC_EstLaneC1R_rad : Inport  Port=5
  VDINR_LaneC2R_rat : Inport  Port=6
  VLIC_EstLaneC2R_rat : Inport  Port=7
  VDINR_LaneC3R_rat : Inport  Port=8
  VLIC_EstLaneC3R_rat : Inport  Port=9
  VDINR_ViewRangeEndR_m : Inport  Port=10
  VLIC_EstViewRangeEndR_m : Inport  Port=11
  Switch{1,4..7} (5 alike) : Switch  Criteria=u2 ~= 0
  OptLaneC0R : Outport
  OptLaneC1R : Outport  Port=2
  OptLaneC2R : Outport  Port=3
  OptLaneC3R : Outport  Port=4
  OptViewRange_R : Outport  Port=5
  wires:
  VDINR_LaneC0R_m/1 -> Switch4/1
  VLIC_EstLaneC0R_m/1 -> Switch4/3
  VDINR_LaneC1R_rad/1 -> Switch5/1
  VLIC_EstLaneC1R_rad/1 -> Switch5/3
  VDINR_LaneC2R_rat/1 -> Switch6/1
  VLIC_EstLaneC2R_rat/1 -> Switch6/3
  Switch6/1 -> OptLaneC2R/1  "OptLaneC2R"
  VDINR_LaneC3R_rat/1 -> Switch7/1
  VLIC_EstLaneC3R_rat/1 -> Switch7/3
  Switch7/1 -> OptLaneC3R/1  "OptLaneC3R"
  Switch4/1 -> OptLaneC0R/1  "OptLaneC0R"
  Switch5/1 -> OptLaneC1R/1  "OptLaneC1R"
  VDINR_ViewRangeEndR_m/1 -> Switch1/1
  UsingRawLaneR_flg/1 -> Switch4/2, Switch6/2, Switch7/2, Switch1/2, Switch5/2
  VLIC_EstViewRangeEndR_m/1 -> Switch1/3
  Switch1/1 -> OptViewRange_R/1  "OptViewRange_R"

== stateflow chart lic_old/Lane_Process/LaneCalculation/Lane_status ==
  (default) -> (junction 9)
  (junction 9) -> (junction 10) [order 1] : [VLIC_LeftLaneAvail_fig && VLIC_RightLaneAvail_fig]
  (junction 9) -> (junction 16) [order 2]
  (junction 10) -> (junction 12) : {SWCase=1;
      | LR_avail=TRUE;
      | R_avail=FALSE;
      | L_avail=FALSE;
      | NO_avail=FALSE;}
  (junction 16) -> (junction 18) [order 1] : [(!VLIC_C2Diff_flg || !VLIC_LeftLaneAvail_fig) && VLIC_RightLaneAvail_fig]
  (junction 16) -> (junction 22) [order 2]
  (junction 18) -> (junction 20) : {SWCase=2;
      | LR_avail=FALSE;
      | R_avail=TRUE;
      | L_avail=FALSE;
      | NO_avail=FALSE;}
  (junction 22) -> (junction 24) [order 1] : [VLIC_LeftLaneAvail_fig && (VLIC_C2Diff_flg || !VLIC_RightLaneAvail_fig)]
  (junction 22) -> (junction 34) [order 2] : {SWCase=4;
      | LR_avail=FALSE;
      | R_avail=FALSE;
      | L_avail=FALSE;
      | NO_avail=TRUE;}
  (junction 24) -> (junction 26) : {SWCase=3;
      | LR_avail=FALSE;
      | R_avail=FALSE;
      | L_avail=TRUE;
      | NO_avail=FALSE;}
  (junction 26) -> (junction 34)
  (junction 20) -> (junction 26)
  (junction 12) -> (junction 20)
  data: VLIC_LeftLaneAvail_fig input; VLIC_RightLaneAvail_fig input; SWCase output single; LR_avail output boolean; R_avail output boolean; L_avail output boolean; NO_avail output boolean; TRUE parameter; FALSE parameter; VLIC_C2Diff_flg input

== stateflow chart lic_old/Lane_Process/LaneCalculation/C1R_Bias/Forgetting_factor/FF ==
  state Forget_Factor
    (default) -> (junction 10) : {P=1;
        | C1RBias_new_store = C1RBias_new;
        | P_R = P;
        | C1R_Bias = C1RBias_new_store;}
    Forget_Factor -> (junction 10)
    (junction 10) -> (junction 13) : {C1RBias_new_store = C1RBias_new_store + P*(C1RBias_new - C1RBias_new_store)/(Forget_Factor+P);
        | P = (P-P*P/(Forget_Factor+P))/Forget_Factor;
        | P_R=P;
        | C1R_Bias=C1RBias_new_store;}
  data: C1RBias_new input; P local single; C1RBias_new_store local single; Forget_Factor input; C1R_Bias output single; P_R output single

== stateflow chart lic_old/Lane_Process/LaneCalculation/C1L_Bias/Forgetting_factor/FF ==
  state Forget_Factor
    (default) -> (junction 10) : {P=1;
        | C1LBias_new_store = C1LBias_new;
        | P_L = P;
        | C1L_Bias = C1LBias_new_store;}
    Forget_Factor -> (junction 10)
    (junction 10) -> (junction 13) : {C1LBias_new_store = C1LBias_new_store + P*(C1LBias_new - C1LBias_new_store)/(Forget_Factor+P);
        | P = (P-P*P/(Forget_Factor+P))/Forget_Factor;
        | P_L=P;
        | C1L_Bias=C1LBias_new_store;}
  data: C1LBias_new input; P local single; C1LBias_new_store local single; Forget_Factor input; C1L_Bias output single; P_L output single
